simulink model "dhaouadi2013_test"  (R2025a)
settings: Solver=VariableStepAuto  StartTime=0.0  StopTime=25  FixedStep=0.01  RelTol=1e-3
InitFcn:
  | simstruct_init();
libraries: dhaouadi2013_lib x5, mmuct_lib x1
settings Model: PacingRate=4  Creator=nicolls  LastModifiedBy=nicolls
settings OptimizationCC: DefaultParameterBehavior=Inlined  EnhancedBackFolding=on  PassReuseOutputArgsAs=Individual arguments  ZeroExternalMemoryAtStartup=off  ZeroInternalMemoryAtStartup=off  OptimizeBlockOrder=speed  DifferentSizesBufferReuse=on  OptimizationCustomize=off  EfficientTunableParamExpr=on
settings DebuggingCC: ParameterTunabilityLossMsg=error
settings SFSimCC: MATLABDynamicMemAlloc=off
settings RTWCC: SystemTargetFile=ert.tlc  GenCodeOnly=on  TemplateMakefile=ert_default_tmf  Description=Embedded Coder
settings CodeAppCC: ForceParamTrailComments=on  IgnoreCustomStorageClasses=off  OperatorAnnotations=on  SimulinkDataObjDesc=on  SFDataObjDesc=on  InsertBlockDesc=on
settings ERTTargetCC: ExtModeTransport=0.0  ExtModeStaticAlloc=off  ExtModeMexFile=ext_comm  ExtModeIntrfLevel=Level1  ERTCustomFileTemplate=example_file_process.tlc  TargetLangStandard=C99 (ISO)  GenerateSampleERTMain=on  SupportContinuousTime=on

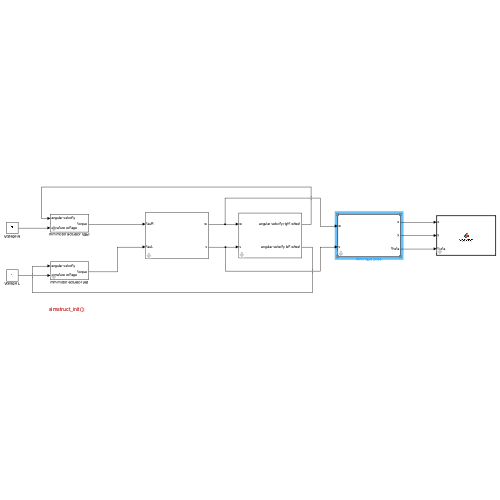
[thumbnail: Simulink's stored preview of the top-level diagram]
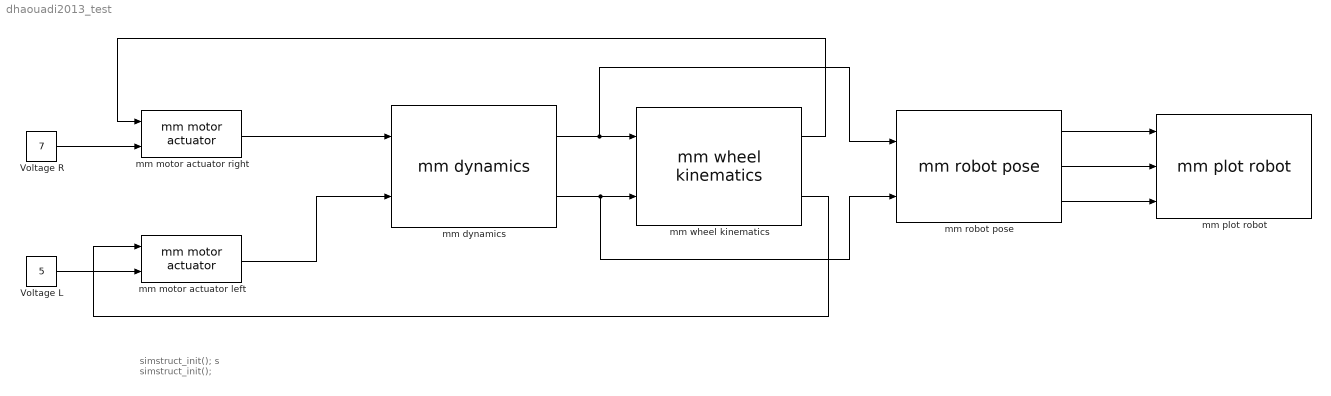
== system dhaouadi2013_test ==
  note: simstruct_init();
      | s
      | simstruct_init();
  Voltage L : Constant  Value=5
  Voltage R : Constant  Value=7
  mm dynamics : dhaouadi2013_lib/mm dynamics  m=5  I=2  L=0.05  d=0  R=0.025  m_c=5  I_w=0
      settings: SourceProductName=UCT dhaouadi2013
  mm motor actuator left : dhaouadi2013_lib/mm motor actuator  La=3  Ra=6  Kb=3  N=2  Kt=2
  mm motor actuator right : dhaouadi2013_lib/mm motor actuator  La=3  Ra=6  Kb=3  N=2  Kt=2
  mm plot robot : mmuct_lib/mm plot robot  simstruct=simstruct  x0=0.1  y0=0.1  theta0=0
      settings: SourceProductName=UCT EEE Micromouse
  mm robot pose : dhaouadi2013_lib/mm robot pose  x0=0.1  y0=0.1  theta0=0
  mm wheel kinematics : dhaouadi2013_lib/mm wheel kinematics  L=0.05  R=0.025
  wires:
  mm wheel kinematics/2 -> mm motor actuator left/1
  Voltage R/1 -> mm motor actuator right/2
  mm motor actuator right/1 -> mm dynamics/1
  mm wheel kinematics/1 -> mm motor actuator right/1
  mm motor actuator left/1 -> mm dynamics/2
  mm dynamics/1 -> mm wheel kinematics/1, mm robot pose/1
  Voltage L/1 -> mm motor actuator left/2
  mm dynamics/2 -> mm wheel kinematics/2, mm robot pose/2
  mm robot pose/1 -> mm plot robot/1
  mm robot pose/2 -> mm plot robot/2
  mm robot pose/3 -> mm plot robot/3
